simulink model "PD_sim"  (R2015a)
settings: Solver=ode45  StartTime=0.0  StopTime=1  RelTol=1e-3
values from neighbouring files (symbols this model uses):
  state_init = zeros(param.Nstates, 1)    [PD_main.m]
undefined symbols (not defined in the file or in its folder): K, param, x, x_dot, y, y_dot
settings Model: Creator=jesus  LastModifiedBy=jesus

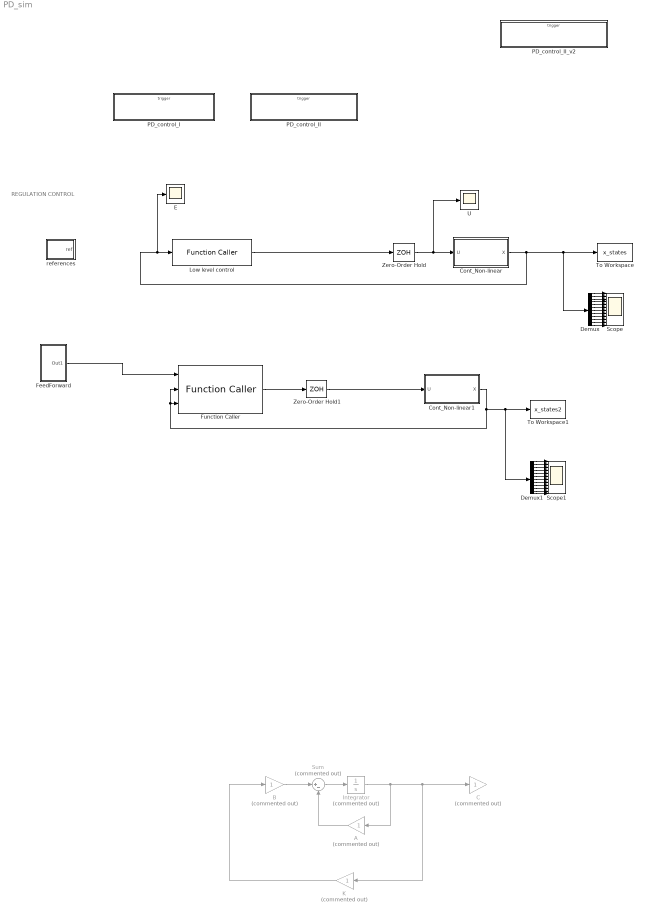
== system PD_sim ==
  note: REGULATION CONTROL
  A : Gain  Commented=on
  B : Gain  Commented=on
  C : Gain  Commented=on
  Cont_Non-linear : Subsystem
  Cont_Non-linear1 : Subsystem
  Demux : Demux  Outputs=12
  Demux1 : Demux  Outputs=12
  E : Scope
      settings: YMin=-1e+08  YMax=1.1e+09  SaveName=ScopeData2
  FeedForward : Subsystem
  Function Caller : FunctionCaller  FunctionPrototype=U = PD_control_II(FF,R,X)
  Integrator : Integrator  Commented=on
  K : Gain  Commented=on
  Low level control : FunctionCaller  FunctionPrototype=U = PD_control(E)
  PD_control_I : Subsystem  TreatAsAtomicUnit=on
  PD_control_II : Subsystem  TreatAsAtomicUnit=on
  PD_control_II_v2 : Subsystem  TreatAsAtomicUnit=on
  Scope : Scope  NumInputPorts=12
      settings: YMin=-8e+08~-5~-5~-5~-5~-5~-5~-5~-5~-5~-5~-5  YMax=1e+08~5~5~5~5~5~5~5~5~5~5~5
  Scope1 : Scope  NumInputPorts=12
      settings: YMin=-8e+08~-5~-5~-5~-5~-5~-5~-5~-5~-5~-5~-5  YMax=1e+08~5~5~5~5~5~5~5~5~5~5~5  SaveName=ScopeData3
  Sum : Sum  Commented=on  Inputs=|+-
  To Workspace : ToWorkspace  VariableName=x_states  SaveFormat=Timeseries  SampleTime=-1
  To Workspace1 : ToWorkspace  VariableName=x_states2  SaveFormat=Timeseries  SampleTime=-1
  U : Scope
      settings: YMin=-1.5e+08  YMax=2.5e+07
  Zero-Order Hold : ZeroOrderHold  SampleTime=param.hs
  Zero-Order Hold1 : ZeroOrderHold  SampleTime=param.hs
  references : Subsystem
  wires:
  Integrator/1 -> A/1, K/1, C/1
  B/1 -> Sum/1
  Sum/1 -> Integrator/1
  A/1 -> Sum/2
  K/1 -> B/1
  Low level control/1 -> Zero-Order Hold/1
  Zero-Order Hold/1 -> Cont_Non-linear/1(U), U/1
  Function Caller/1 -> Zero-Order Hold1/1
  Demux/1 -> Scope/1
  Demux/2 -> Scope/2
  Demux/3 -> Scope/3
  Demux/4 -> Scope/4
  Demux/5 -> Scope/5
  Demux/6 -> Scope/6
  Demux/7 -> Scope/7
  Demux/8 -> Scope/8
  Demux/9 -> Scope/9
  Demux/10 -> Scope/10
  Demux/11 -> Scope/11
  Demux/12 -> Scope/12
  Zero-Order Hold1/1 -> Cont_Non-linear1/1(U)
  FeedForward/1(Out1) -> Function Caller/1
  Cont_Non-linear1/1(X) -> Demux1/1, To Workspace1/1, Function Caller/2, Function Caller/3
  Demux1/3 -> Scope1/3
  Demux1/4 -> Scope1/4
  Demux1/5 -> Scope1/5
  Demux1/6 -> Scope1/6
  Demux1/7 -> Scope1/7
  Demux1/8 -> Scope1/8
  Demux1/9 -> Scope1/9
  Demux1/10 -> Scope1/10
  Demux1/11 -> Scope1/11
  Demux1/12 -> Scope1/12
  Demux1/2 -> Scope1/2
  Demux1/1 -> Scope1/1
  Cont_Non-linear/1(X) -> Low level control/1, E/1, Demux/1, To Workspace/1

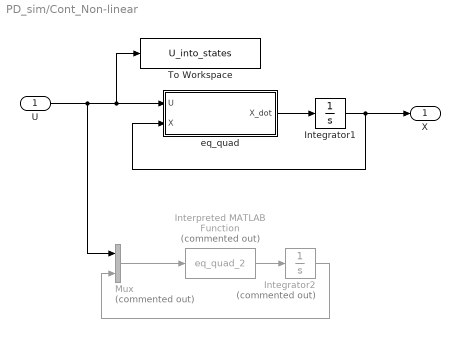
== system PD_sim/Cont_Non-linear ==
  U : Inport
  Integrator1 : Integrator  InitialCondition=state_init
  Integrator2 : Integrator  Commented=on  InitialCondition=state_init
  Interpreted MATLAB Function : MATLABFcn  Commented=on  MATLABFcn=eq_quad_2
  Mux : Mux  Commented=on  Inputs=2
  To Workspace : ToWorkspace  VariableName=U_into_states  SaveFormat=Timeseries  SampleTime=-1
  eq_quad : MATLAB Function  TreatAsAtomicUnit=on
  X : Outport
  wires:
  Integrator1/1 -> X/1, eq_quad/2(X)
  U/1 -> Mux/1, To Workspace/1, eq_quad/1(U)
  eq_quad/1(X_dot) -> Integrator1/1
  Interpreted MATLAB Function/1 -> Integrator2/1
  Mux/1 -> Interpreted MATLAB Function/1
  Integrator2/1 -> Mux/2

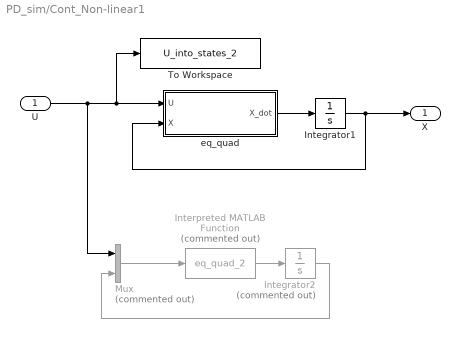
== system PD_sim/Cont_Non-linear1 ==
  U : Inport
  Integrator1 : Integrator  InitialCondition=state_init
  Integrator2 : Integrator  Commented=on  InitialCondition=state_init
  Interpreted MATLAB Function : MATLABFcn  Commented=on  MATLABFcn=eq_quad_2
  Mux : Mux  Commented=on  Inputs=2
  To Workspace : ToWorkspace  VariableName=U_into_states_2  SaveFormat=Timeseries  SampleTime=-1
  eq_quad : MATLAB Function  TreatAsAtomicUnit=on
  X : Outport
  wires:
  Integrator1/1 -> X/1, eq_quad/2(X)
  U/1 -> Mux/1, To Workspace/1, eq_quad/1(U)
  eq_quad/1(X_dot) -> Integrator1/1
  Interpreted MATLAB Function/1 -> Integrator2/1
  Mux/1 -> Interpreted MATLAB Function/1
  Integrator2/1 -> Mux/2

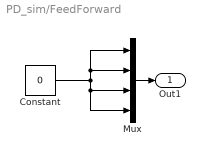
== system PD_sim/FeedForward ==
  Constant : Constant  Value=0
  Mux : Mux
  Out1 : Outport
  wires:
  Constant/1 -> Mux/4, Mux/3, Mux/1, Mux/2
  Mux/1 -> Out1/1

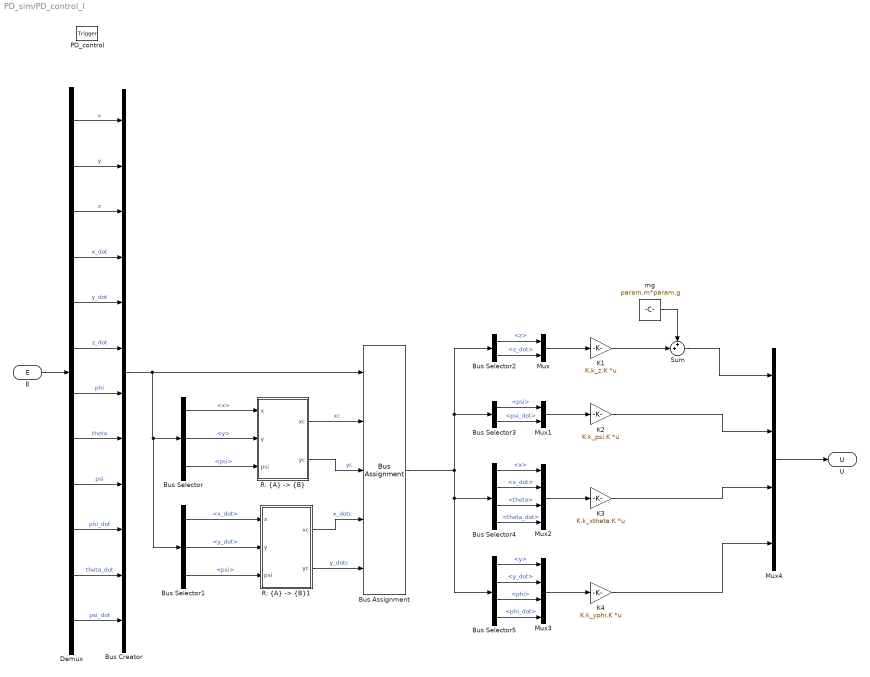
== system PD_sim/PD_control_I ==
  PD_control : TriggerPort  TriggerType=function-call  IsSimulinkFunction=on  FunctionName=PD_control
  Bus Assignment : BusAssignment  AssignedSignals=x,y,x_dot,y_dot
  Bus Creator : BusCreator  Inputs=12
  Bus Selector : BusSelector  OutputSignals=x,y,psi
  Bus Selector1 : BusSelector  OutputSignals=x_dot,y_dot,psi
  Bus Selector2 : BusSelector  OutputSignals=z,z_dot
  Bus Selector3 : BusSelector  OutputSignals=psi,psi_dot
  Bus Selector4 : BusSelector  OutputSignals=x,x_dot,theta,theta_dot
  Bus Selector5 : BusSelector  OutputSignals=y,y_dot,phi,phi_dot
  Demux : Demux  Outputs=12
  K1 : Gain  Gain=K.k_z.K  Multiplication=Matrix(K*u)
  K2 : Gain  Gain=K.k_psi.K  Multiplication=Matrix(K*u)
  K3 : Gain  Gain=K.k_xtheta.K  Multiplication=Matrix(K*u)
  K4 : Gain  Gain=K.k_yphi.K  Multiplication=Matrix(K*u)
  Mux : Mux  Inputs=2
  Mux1 : Mux  Inputs=2
  Mux2 : Mux
  Mux3 : Mux
  Mux4 : Mux
  "R: {A} -> {B}" : MATLAB Function  TreatAsAtomicUnit=on
  "R: {A} -> {B}1" : MATLAB Function  TreatAsAtomicUnit=on
  Sum : Sum  Inputs=++|
  mg : Constant  Value=param.m*param.g  SampleTime=-1
  E : ArgIn  DisableCoverage=on  PortDimensions=12  ArgumentName=E
  U : ArgOut  DisableCoverage=on  PortDimensions=4  ArgumentName=U
  wires:
  E/1 -> Demux/1
  Demux/1 -> Bus Creator/1  "x"
  Demux/2 -> Bus Creator/2  "y"
  Demux/12 -> Bus Creator/12  "psi_dot"
  Demux/7 -> Bus Creator/7  "phi"
  Demux/8 -> Bus Creator/8  "theta"
  Demux/3 -> Bus Creator/3  "z"
  Demux/4 -> Bus Creator/4  "x_dot"
  Demux/5 -> Bus Creator/5  "y_dot"
  Demux/6 -> Bus Creator/6  "z_dot"
  Demux/9 -> Bus Creator/9  "psi"
  Demux/10 -> Bus Creator/10  "phi_dot"
  Demux/11 -> Bus Creator/11  "theta_dot"
  Bus Selector/1 -> "R: {A} -> {B}"/1(x)  "<x>"
  Bus Selector/2 -> "R: {A} -> {B}"/2(y)  "<y>"
  Bus Selector/3 -> "R: {A} -> {B}"/3(psi)  "<psi>"
  "R: {A} -> {B}"/1(xc) -> Bus Assignment/2  "xc"
  "R: {A} -> {B}"/2(yc) -> Bus Assignment/3  "yc"
  Bus Creator/1 -> Bus Assignment/1, Bus Selector1/1, Bus Selector/1
  Bus Selector1/1 -> "R: {A} -> {B}1"/1(x)  "<x_dot>"
  Bus Selector1/2 -> "R: {A} -> {B}1"/2(y)  "<y_dot>"
  Bus Selector1/3 -> "R: {A} -> {B}1"/3(psi)  "<psi>"
  "R: {A} -> {B}1"/1(xc) -> Bus Assignment/4  "x_dotc"
  "R: {A} -> {B}1"/2(yc) -> Bus Assignment/5  "y_dotc"
  Bus Assignment/1 -> Bus Selector2/1, Bus Selector3/1, Bus Selector5/1, Bus Selector4/1
  Bus Selector2/1 -> Mux/1  "<z>"
  Bus Selector2/2 -> Mux/2  "<z_dot>"
  Bus Selector3/1 -> Mux1/1  "<psi>"
  Bus Selector3/2 -> Mux1/2  "<psi_dot>"
  Bus Selector5/1 -> Mux3/1  "<y>"
  Bus Selector5/2 -> Mux3/2  "<y_dot>"
  Bus Selector5/3 -> Mux3/3  "<phi>"
  Bus Selector5/4 -> Mux3/4  "<phi_dot>"
  Bus Selector4/4 -> Mux2/4  "<theta_dot>"
  Bus Selector4/3 -> Mux2/3  "<theta>"
  Bus Selector4/2 -> Mux2/2  "<x_dot>"
  Bus Selector4/1 -> Mux2/1  "<x>"
  Mux2/1 -> K3/1
  Mux1/1 -> K2/1
  Mux/1 -> K1/1
  Mux3/1 -> K4/1
  Mux4/1 -> U/1
  K3/1 -> Mux4/3
  K2/1 -> Mux4/2
  K4/1 -> Mux4/4
  Sum/1 -> Mux4/1
  K1/1 -> Sum/2
  mg/1 -> Sum/1

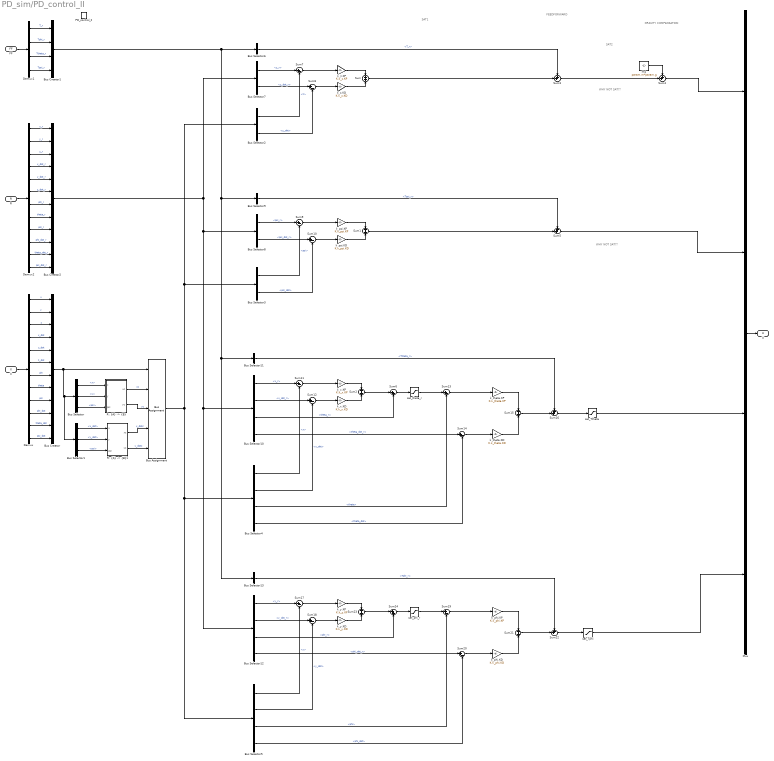
== system PD_sim/PD_control_II ==
  note: WHY NOT SAT??
  note: WHY NOT SAT??
  note: SAT2
  note: SAT1
  note: FEEDFORWARD
  note: GRAVITY
      | COMPENSATION
  PD_control_II : TriggerPort  TriggerType=function-call  IsSimulinkFunction=on  FunctionName=PD_control_II
  Bus Assignment : BusAssignment  AssignedSignals=x,y,x_dot,y_dot
  Bus Creator : BusCreator  Inputs=12
  Bus Creator1 : BusCreator
  Bus Creator2 : BusCreator  Inputs=12
  Bus Selector : BusSelector  OutputSignals=x,y,psi
  Bus Selector1 : BusSelector  OutputSignals=x_dot,y_dot,psi
  Bus Selector10 : BusSelector  OutputSignals=x_r,x_dot_r,theta_r,theta_dot_r
  Bus Selector11 : BusSelector  OutputSignals=Ttheta_r
  Bus Selector12 : BusSelector  OutputSignals=y_r,y_dot_r,phi_r,phi_dot_r
  Bus Selector13 : BusSelector  OutputSignals=Tphi_r
  Bus Selector2 : BusSelector  OutputSignals=z,z_dot
  Bus Selector3 : BusSelector  OutputSignals=psi,psi_dot
  Bus Selector4 : BusSelector  OutputSignals=x,x_dot,theta,theta_dot
  Bus Selector5 : BusSelector  OutputSignals=y,y_dot,phi,phi_dot
  Bus Selector6 : BusSelector  OutputSignals=T_r
  Bus Selector7 : BusSelector  OutputSignals=z_r,z_dot_r
  Bus Selector8 : BusSelector  OutputSignals=psi_r,psi_dot_r
  Bus Selector9 : BusSelector  OutputSignals=Tpsi_r
  Demux : Demux  Outputs=12
  Demux1 : Demux
  Demux2 : Demux  Outputs=12
  Mux : Mux
  "R: {A} -> {B}" : MATLAB Function  TreatAsAtomicUnit=on
  "R: {A} -> {B}1" : MATLAB Function  TreatAsAtomicUnit=on
  Sum{,1..2,15,21,23} (6 alike) : Sum  Inputs=+|+
  Sum{7..14,17..20} (12 alike) : Sum  Inputs=|+-
  Sum{3..5,16,22} (5 alike) : Sum  Inputs=++|
  Sum24 : Sum  Inputs=|++
  Sum6 : Sum  Inputs=|++
  k_phi.KD : Gain  Gain=K.k_phi.KD
  k_phi.KP : Gain  Gain=K.k_phi.KP
  k_psi.KD : Gain  Gain=K.k_psi.KD
  k_psi.KP : Gain  Gain=K.k_psi.KP
  k_theta.KD : Gain  Gain=K.k_theta.KD
  k_theta.KP : Gain  Gain=K.k_theta.KP
  k_x.KD : Gain  Gain=K.k_x.KD
  k_x.KP : Gain  Gain=K.k_x.KP
  k_y.KD : Gain  Gain=K.k_y.KD
  k_y.KP : Gain  Gain=K.k_y.KP
  k_z.KD : Gain  Gain=K.k_z.KD
  k_z.KP : Gain  Gain=K.k_z.KP
  mg : Constant  Value=param.m*param.g
  sat_Tphi : Saturate  UpperLimit=param.sat.Tphi.max  LowerLimit=param.sat.Tphi.min
  sat_Ttheta : Saturate  UpperLimit=param.sat.Ttheta.max  LowerLimit=param.sat.Ttheta.min
  sat_phi_r : Saturate  UpperLimit=param.sat.phi_r.max  LowerLimit=param.sat.phi_r.min
  sat_theta_r : Saturate  UpperLimit=param.sat.theta_r.max  LowerLimit=param.sat.theta_r.min
  FF : ArgIn  DisableCoverage=on  PortDimensions=4  ArgumentName=FF
  R : ArgIn  Port=2  PortDimensions=12  ArgumentName=R
  X : ArgIn  Port=3  PortDimensions=12  ArgumentName=X
  U : ArgOut  DisableCoverage=on  PortDimensions=4  ArgumentName=U
  wires:
  Demux/1 -> Bus Creator/1  "x"
  Demux/2 -> Bus Creator/2  "y"
  Demux/3 -> Bus Creator/3  "z"
  Demux/4 -> Bus Creator/4  "x_dot"
  Demux/5 -> Bus Creator/5  "y_dot"
  Demux/6 -> Bus Creator/6  "z_dot"
  Demux/7 -> Bus Creator/7  "phi"
  Demux/8 -> Bus Creator/8  "theta"
  Demux/9 -> Bus Creator/9  "psi"
  Demux/10 -> Bus Creator/10  "phi_dot"
  Demux/11 -> Bus Creator/11  "theta_dot"
  Demux/12 -> Bus Creator/12  "psi_dot"
  Bus Selector/1 -> "R: {A} -> {B}"/1(x)  "<x>"
  Bus Selector/2 -> "R: {A} -> {B}"/2(y)  "<y>"
  Bus Selector/3 -> "R: {A} -> {B}"/3(psi)  "<psi>"
  "R: {A} -> {B}"/1(xc) -> Bus Assignment/2  "xc"
  "R: {A} -> {B}"/2(yc) -> Bus Assignment/3  "yc"
  Bus Creator/1 -> Bus Assignment/1, Bus Selector1/1, Bus Selector/1
  Bus Selector1/1 -> "R: {A} -> {B}1"/1(x)  "<x_dot>"
  Bus Selector1/2 -> "R: {A} -> {B}1"/2(y)  "<y_dot>"
  Bus Selector1/3 -> "R: {A} -> {B}1"/3(psi)  "<psi>"
  "R: {A} -> {B}1"/1(xc) -> Bus Assignment/4  "x_dotc"
  "R: {A} -> {B}1"/2(yc) -> Bus Assignment/5  "y_dotc"
  Bus Assignment/1 -> Bus Selector4/1, Bus Selector5/1, Bus Selector2/1, Bus Selector3/1
  Demux1/1 -> Bus Creator1/1  "T_r"
  Demux1/2 -> Bus Creator1/2  "Tphi_r"
  Demux1/3 -> Bus Creator1/3  "Ttheta_r"
  Demux1/4 -> Bus Creator1/4  "Tpsi_r"
  k_psi.KP/1 -> Sum1/1
  k_psi.KD/1 -> Sum1/2
  k_x.KP/1 -> Sum2/1
  k_x.KD/1 -> Sum2/2
  Sum/1 -> Sum3/2
  Sum3/1 -> Sum4/2
  mg/1 -> Sum4/1
  Sum1/1 -> Sum5/2
  Sum6/1 -> sat_theta_r/1
  X/1 -> Demux/1
  FF/1 -> Demux1/1
  R/1 -> Demux2/1
  Demux2/1 -> Bus Creator2/1  "x_r"
  Demux2/2 -> Bus Creator2/2  "y_r"
  Demux2/3 -> Bus Creator2/3  "z_r"
  Demux2/4 -> Bus Creator2/4  "x_dot_r"
  Demux2/5 -> Bus Creator2/5  "y_dot_r"
  Demux2/6 -> Bus Creator2/6  "z_dot_r"
  Demux2/7 -> Bus Creator2/7  "phi_r"
  Demux2/8 -> Bus Creator2/8  "theta_r"
  Demux2/9 -> Bus Creator2/9  "psi_r"
  Demux2/10 -> Bus Creator2/10  "phi_dot_r"
  Demux2/11 -> Bus Creator2/11  "theta_dot_r"
  Demux2/12 -> Bus Creator2/12  "psi_dot_r"
  Bus Creator2/1 -> Bus Selector12/1, Bus Selector10/1, Bus Selector8/1, Bus Selector7/1
  Bus Selector2/1 -> Sum7/2  "<z>"
  Bus Selector2/2 -> Sum8/2  "<z_dot>"
  Bus Selector7/1 -> Sum7/1  "<z_r>"
  Bus Selector7/2 -> Sum8/1  "<z_dot_r>"
  Sum8/1 -> k_z.KD/1
  Sum7/1 -> k_z.KP/1
  k_z.KP/1 -> Sum/1
  k_z.KD/1 -> Sum/2
  Bus Creator1/1 -> Bus Selector13/1, Bus Selector11/1, Bus Selector9/1, Bus Selector6/1
  Bus Selector6/1 -> Sum3/1  "<T_r>"
  Bus Selector3/1 -> Sum9/2  "<psi>"
  Bus Selector3/2 -> Sum10/2  "<psi_dot>"
  Bus Selector8/1 -> Sum9/1  "<psi_r>"
  Bus Selector8/2 -> Sum10/1  "<psi_dot_r>"
  Bus Selector9/1 -> Sum5/1  "<Tpsi_r>"
  Sum10/1 -> k_psi.KD/1
  Sum9/1 -> k_psi.KP/1
  Bus Selector4/1 -> Sum11/2  "<x>"
  Bus Selector4/2 -> Sum12/2  "<x_dot>"
  Bus Selector4/3 -> Sum13/2  "<theta>"
  Bus Selector4/4 -> Sum14/2  "<theta_dot>"
  Bus Selector10/1 -> Sum11/1  "<x_r>"
  Bus Selector10/2 -> Sum12/1  "<x_dot_r>"
  Bus Selector10/3 -> Sum6/2  "<theta_r>"
  Bus Selector10/4 -> Sum14/1  "<theta_dot_r>"
  Sum12/1 -> k_x.KD/1
  Sum11/1 -> k_x.KP/1
  Sum2/1 -> Sum6/1
  sat_theta_r/1 -> Sum13/1
  Sum14/1 -> k_theta.KD/1
  Sum13/1 -> k_theta.KP/1
  k_theta.KP/1 -> Sum15/1
  k_theta.KD/1 -> Sum15/2
  Sum15/1 -> Sum16/2
  Bus Selector11/1 -> Sum16/1  "<Ttheta_r>"
  k_y.KP/1 -> Sum23/1
  k_y.KD/1 -> Sum23/2
  Sum24/1 -> sat_phi_r/1
  Bus Selector5/1 -> Sum17/2  "<y>"
  Bus Selector5/2 -> Sum18/2  "<y_dot>"
  Bus Selector5/3 -> Sum19/2  "<phi>"
  Bus Selector5/4 -> Sum20/2  "<phi_dot>"
  Bus Selector12/1 -> Sum17/1  "<y_r>"
  Bus Selector12/2 -> Sum18/1  "<y_dot_r>"
  Bus Selector12/3 -> Sum24/2  "<phi_r>"
  Bus Selector12/4 -> Sum20/1  "<phi_dot_r>"
  Sum18/1 -> k_y.KD/1
  Sum17/1 -> k_y.KP/1
  Sum23/1 -> Sum24/1
  sat_phi_r/1 -> Sum19/1
  Sum20/1 -> k_phi.KD/1
  Sum19/1 -> k_phi.KP/1
  k_phi.KP/1 -> Sum21/1
  k_phi.KD/1 -> Sum21/2
  Sum21/1 -> Sum22/2
  Bus Selector13/1 -> Sum22/1  "<Tphi_r>"
  Mux/1 -> U/1
  Sum22/1 -> sat_Tphi/1
  Sum16/1 -> sat_Ttheta/1
  Sum4/1 -> Mux/1
  Sum5/1 -> Mux/2
  sat_Ttheta/1 -> Mux/3
  sat_Tphi/1 -> Mux/4

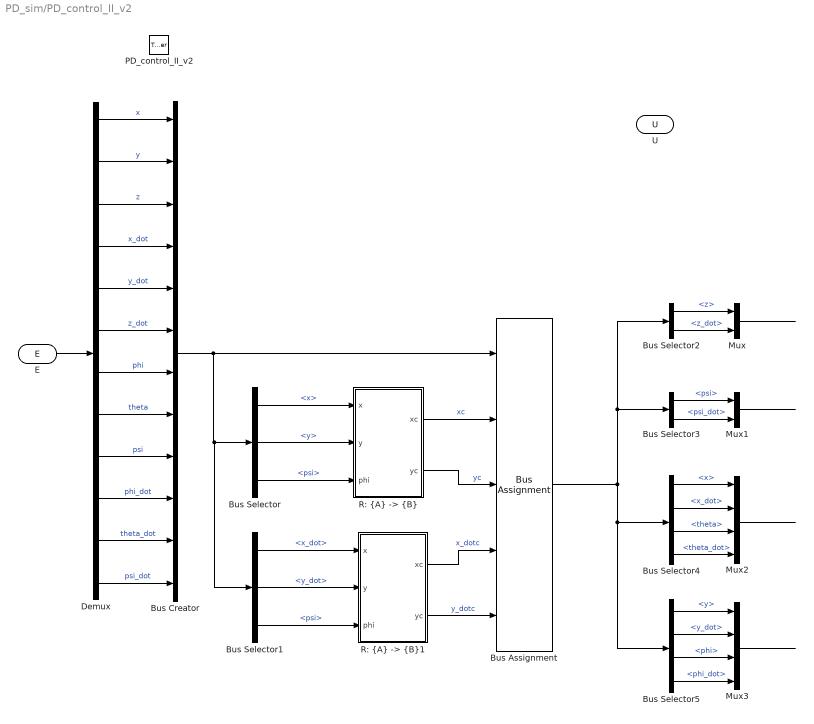
== system PD_sim/PD_control_II_v2 ==
  PD_control_II_v2 : TriggerPort  TriggerType=function-call  IsSimulinkFunction=on  FunctionName=PD_control_II_v2
  Bus Assignment : BusAssignment  AssignedSignals=x,y,x_dot,y_dot
  Bus Creator : BusCreator  Inputs=12
  Bus Selector : BusSelector  OutputSignals=x,y,psi
  Bus Selector1 : BusSelector  OutputSignals=x_dot,y_dot,psi
  Bus Selector2 : BusSelector  OutputSignals=z,z_dot
  Bus Selector3 : BusSelector  OutputSignals=psi,psi_dot
  Bus Selector4 : BusSelector  OutputSignals=x,x_dot,theta,theta_dot
  Bus Selector5 : BusSelector  OutputSignals=y,y_dot,phi,phi_dot
  Demux : Demux  Outputs=12
  Mux : Mux  Inputs=2
  Mux1 : Mux  Inputs=2
  Mux2 : Mux
  Mux3 : Mux
  "R: {A} -> {B}" : MATLAB Function  TreatAsAtomicUnit=on
  "R: {A} -> {B}1" : MATLAB Function  TreatAsAtomicUnit=on
  E : ArgIn  DisableCoverage=on  PortDimensions=12  ArgumentName=E
  U : ArgOut  DisableCoverage=on  ArgumentName=U
  wires:
  E/1 -> Demux/1
  Demux/1 -> Bus Creator/1  "x"
  Demux/2 -> Bus Creator/2  "y"
  Demux/3 -> Bus Creator/3  "z"
  Demux/4 -> Bus Creator/4  "x_dot"
  Demux/5 -> Bus Creator/5  "y_dot"
  Demux/6 -> Bus Creator/6  "z_dot"
  Demux/7 -> Bus Creator/7  "phi"
  Demux/8 -> Bus Creator/8  "theta"
  Demux/9 -> Bus Creator/9  "psi"
  Demux/10 -> Bus Creator/10  "phi_dot"
  Demux/11 -> Bus Creator/11  "theta_dot"
  Demux/12 -> Bus Creator/12  "psi_dot"
  Bus Selector/1 -> "R: {A} -> {B}"/1(x)  "<x>"
  Bus Selector/2 -> "R: {A} -> {B}"/2(y)  "<y>"
  Bus Selector/3 -> "R: {A} -> {B}"/3(phi)  "<psi>"
  "R: {A} -> {B}"/1(xc) -> Bus Assignment/2  "xc"
  "R: {A} -> {B}"/2(yc) -> Bus Assignment/3  "yc"
  Bus Creator/1 -> Bus Assignment/1, Bus Selector1/1, Bus Selector/1
  Bus Selector1/1 -> "R: {A} -> {B}1"/1(x)  "<x_dot>"
  Bus Selector1/2 -> "R: {A} -> {B}1"/2(y)  "<y_dot>"
  Bus Selector1/3 -> "R: {A} -> {B}1"/3(phi)  "<psi>"
  "R: {A} -> {B}1"/1(xc) -> Bus Assignment/4  "x_dotc"
  "R: {A} -> {B}1"/2(yc) -> Bus Assignment/5  "y_dotc"
  Bus Assignment/1 -> Bus Selector2/1, Bus Selector3/1, Bus Selector5/1, Bus Selector4/1
  Bus Selector2/1 -> Mux/1  "<z>"
  Bus Selector2/2 -> Mux/2  "<z_dot>"
  Bus Selector3/1 -> Mux1/1  "<psi>"
  Bus Selector3/2 -> Mux1/2  "<psi_dot>"
  Bus Selector5/1 -> Mux3/1  "<y>"
  Bus Selector5/2 -> Mux3/2  "<y_dot>"
  Bus Selector5/3 -> Mux3/3  "<phi>"
  Bus Selector5/4 -> Mux3/4  "<phi_dot>"
  Bus Selector4/4 -> Mux2/4  "<theta_dot>"
  Bus Selector4/3 -> Mux2/3  "<theta>"
  Bus Selector4/2 -> Mux2/2  "<x_dot>"
  Bus Selector4/1 -> Mux2/1  "<x>"
  Mux2/1 -> ?
  Mux1/1 -> ?
  Mux/1 -> ?
  Mux3/1 -> ?

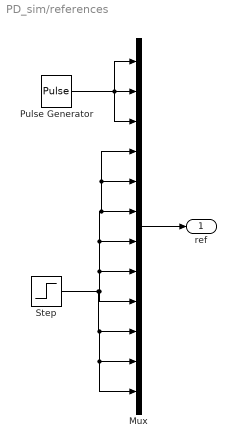
== system PD_sim/references ==
  Mux : Mux  Inputs=param.Nstates
  Pulse Generator : DiscretePulseGenerator  PulseType=Time based  Period=6  PulseWidth=50
  Step : Step  Time=10  SampleTime=0
  ref : Outport
  wires:
  Mux/1 -> ref/1
  Pulse Generator/1 -> Mux/3, Mux/1, Mux/2
  Step/1 -> Mux/12, Mux/11, Mux/10, Mux/4, Mux/5, Mux/6, Mux/7, Mux/8, Mux/9

== matlab function PD_sim/PD_control_I/R: {A} -> {B} ==
  data: x input; y input; psi input; xc output; yc output
function [xc, yc] = fcn(x, y, psi)
%#codegen
% Change in cordenates from fixed frame {A} to body frame {B} of position
%  state coordenates
% · apply rotation matrix over phi (vertical) to [x] and [y]
% · the references are given in fix frame {A}, input [u] is computed in
%   body frame {B}

R = [ cos(psi) sin(psi)
     -sin(psi) cos(psi)];
a = R * [x, y]';
xc = a(1);
yc = a(2);

== matlab function PD_sim/Cont_Non-linear/eq_quad ==
  data: U input; X input; X_dot output
function X_dot = f(U, X)
% %#codegen
% State
    x      = X(1);     Vx   = X(4);
    y      = X(2);     Vy   = X(5);
    z      = X(3);     Vz   = X(6);

    phi    = X(7);     p    = X(10);
    theta  = X(8);     q    = X(11);
    psi    = X(9);     r    = X(12);

% Inputs
    T  = U(1);       Tphi   = U(2);
                     Ttheta = U(3);
                     Tpsi   = U(4);
                     
% Parameters
    %global param
%     m  = param.m;    g = param.g;
%     Ix = param.Ix;  Iy = param.Iy;  Iz = param.Iz;
    m=0.429;    g=9.8067;
    Ix=0.0022;  Iy=0.0030;  Iz=0.0048;
    Nstates=12;
% Equations
X_dot = zeros(Nstates, 1);

X_dot(1)  = Vx;
X_dot(2)  = Vy;
X_dot(3)  = Vz;

X_dot(4)  = -(T/m) * ( sin(theta)*sin(psi) + cos(phi)*sin(theta)*cos(psi) );
X_dot(5)  = -(T/m) * ( cos(phi)*sin(theta)*sin(psi) - sin(phi)*cos(psi) );
X_dot(6)  = -(T/m) * ( cos(phi)*cos(theta) ) + g;

X_dot(7)  = p + sin(phi)*tan(theta)*q + ( cos(phi)*tan(theta) )*r;
X_dot(8)  = cos(phi)*q - sin(phi)*r;
X_dot(9)  = ( sin(phi)/cos(theta) )*q + ( cos(phi)/cos(theta) )*r;

X_dot(10) = ( (Iy-Iz)/Ix )*r*q + Tphi   / Ix;
X_dot(11) = ( (Iz-Ix)/Iy )*p*r + Ttheta / Iy;
X_dot(12) = ( (Ix-Iy)/Iz )*p*q + Tpsi   / Iz;

% states as a column vector
% x_dot = x_dot';

== matlab function PD_sim/PD_control_I/R: {A} -> {B}1 ==
  data: x input; y input; psi input; xc output; yc output
function [xc, yc] = fcn(x, y, psi)
%#codegen
% Change in cordenates from fixed frame {A} to body frame {B} of position
%  state coordenates
% · apply rotation matrix over phi (vertical) to [x] and [y]
% · the references are given in fix frame {A}, input [u] is computed in
%   body frame {B}

R = [ cos(psi) sin(psi)
     -sin(psi) cos(psi)];
a = R * [x; y];
xc = a(1); 
yc = a(2);

== matlab function PD_sim/PD_control_II/R: {A} -> {B} ==
  data: x input; y input; psi input; xc output; yc output
function [xc, yc] = fcn(x, y, psi)
%#codegen
% Change in cordenates from fixed frame {A} to body frame {B} of position
%  state coordenates
% · apply rotation matrix over phi (vertical) to [x] and [y]
% · the references are given in fix frame {A}, input [u] is computed in
%   body frame {B}

R = [ cos(psi) sin(psi)
     -sin(psi) cos(psi)];
a = R * [x, y]';
xc = a(1);
yc = a(2);

== matlab function PD_sim/PD_control_II/R: {A} -> {B}1 ==
  data: x input; y input; psi input; xc output; yc output
function [xc, yc] = fcn(x, y, psi)
%#codegen
% Change in cordenates from fixed frame {A} to body frame {B} of position
%  state coordenates
% · apply rotation matrix over phi (vertical) to [x] and [y]
% · the references are given in fix frame {A}, input [u] is computed in
%   body frame {B}

R = [ cos(psi) sin(psi)
     -sin(psi) cos(psi)];
a = R * [x; y];
xc = a(1); 
yc = a(2);

== matlab function PD_sim/PD_control_II_v2/R: {A} -> {B} ==
  data: x input; y input; phi input; xc output; yc output
function [xc, yc] = fcn(x, y, phi)
%#codegen
% Change in cordenates from fixed frame {A} to body frame {B} of position
%  state coordenates
% · apply rotation matrix over phi (vertical) to [x] and [y]
% · the references are given in fix frame {A}, input [u] is computed in
%   body frame {B}

R = [ cos(phi) sin(phi)
     -sin(phi) cos(phi)];
a = R * [x, y]';
xc = a(1);
yc = a(2);

== matlab function PD_sim/PD_control_II_v2/R: {A} -> {B}1 ==
  data: x input; y input; phi input; xc output; yc output
function [xc, yc] = fcn(x, y, phi)
%#codegen
% Change in cordenates from fixed frame {A} to body frame {B} of position
%  state coordenates
% · apply rotation matrix over phi (vertical) to [x] and [y]
% · the references are given in fix frame {A}, input [u] is computed in
%   body frame {B}

R = [ cos(phi) sin(phi)
     -sin(phi) cos(phi)];
a = R * [x; y];
xc = a(1); 
yc = a(2);

== matlab function PD_sim/Cont_Non-linear1/eq_quad ==
  data: U input; X input; X_dot output
function X_dot = f(U, X)
% %#codegen
% State
    x      = X(1);     Vx   = X(4);
    y      = X(2);     Vy   = X(5);
    z      = X(3);     Vz   = X(6);

    phi    = X(7);     p    = X(10);
    theta  = X(8);     q    = X(11);
    psi    = X(9);     r    = X(12);

% Inputs
    T  = U(1);       Tphi   = U(2);
                     Ttheta = U(3);
                     Tpsi   = U(4);
                     
% Parameters
    %global param
%     m  = param.m;    g = param.g;
%     Ix = param.Ix;  Iy = param.Iy;  Iz = param.Iz;
    m=0.429;    g=9.8067;
    Ix=0.0022;  Iy=0.0030;  Iz=0.0048;
    Nstates=12;
% Equations
X_dot = zeros(Nstates, 1);

X_dot(1)  = Vx;
X_dot(2)  = Vy;
X_dot(3)  = Vz;

X_dot(4)  = -(T/m) * ( sin(theta)*sin(psi) + cos(phi)*sin(theta)*cos(psi) );
X_dot(5)  = -(T/m) * ( cos(phi)*sin(theta)*sin(psi) - sin(phi)*cos(psi) );
X_dot(6)  = -(T/m) * ( cos(phi)*cos(theta) ) + g;

X_dot(7)  = p + sin(phi)*tan(theta)*q + ( cos(phi)*tan(theta) )*r;
X_dot(8)  = cos(phi)*q - sin(phi)*r;
X_dot(9)  = ( sin(phi)/cos(theta) )*q + ( cos(phi)/cos(theta) )*r;

X_dot(10) = ( (Iy-Iz)/Ix )*r*q + Tphi   / Ix;
X_dot(11) = ( (Iz-Ix)/Iy )*p*r + Ttheta / Iy;
X_dot(12) = ( (Ix-Iy)/Iz )*p*q + Tpsi   / Iz;

% states as a column vector
% x_dot = x_dot';
